simulink model "req1"  (R2019a)
settings: Solver=FixedStepAuto  StartTime=0.0  StopTime=100  RelTol=1e-3
libraries: sldvlib x1
settings Model: Creator=e40014285  LastModifiedBy=e40014285
settings ConfigComp: CovEnable=on  RecordCoverage=on  CovHtmlReporting=on  CovCumulativeReport=on  CovModelRefEnable=on  DVModelCoverageObjectives=MCDC  DVTestSuiteOptimization=Auto  DVDetectOutOfBounds=on  DVRebuildModelRepresentation=Always

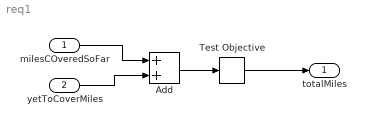
== system req1 ==
  milesCOveredSoFar : Inport  OutDataTypeStr=double
  yetToCoverMiles : Inport  Port=2  OutDataTypeStr=double
  Add : Sum
  Test Objective : sldvlib/Objectives and Constraints/Test Objective  enabled=on  customAVTBlockType=Test Objective  intervals={0,1}  dispValues=on  outEnabled=on
      settings: AttributesFormatString=%<intervals>  SourceProductName=Simulink  SourceProductBaseCode=SL
  totalMiles : Outport  OutDataTypeStr=double
  wires:
  yetToCoverMiles/1 -> Add/2
  milesCOveredSoFar/1 -> Add/1
  Add/1 -> Test Objective/1
  Test Objective/1 -> totalMiles/1
